simulink subsystem "sensorModel"  (R2021a)
settings: Solver=VariableStepAuto  StartTime=0.0  StopTime=10.0  RelTol=1e-3
settings Model: Creator=Laura  LastModifiedBy=Laura

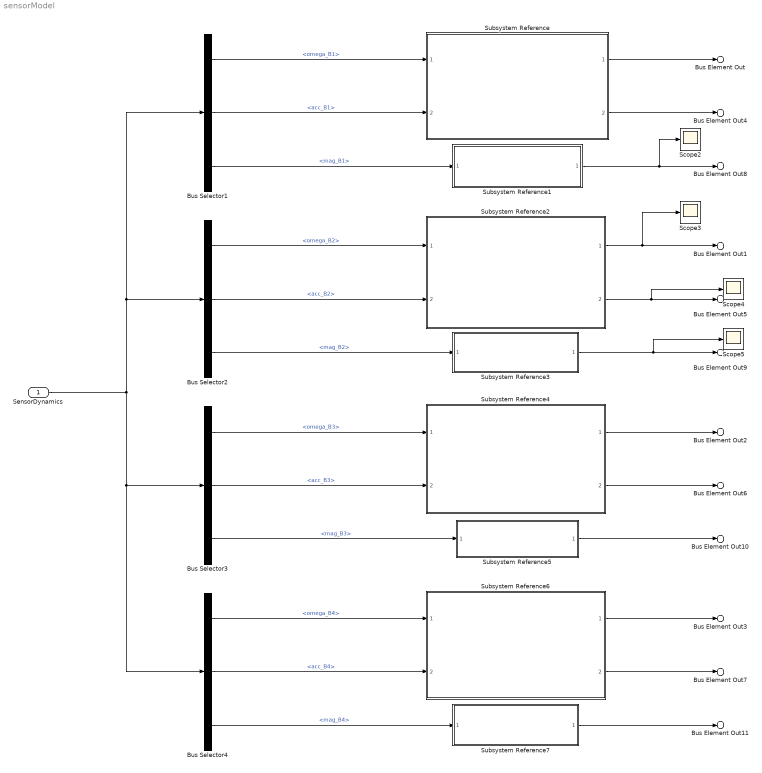
== system sensorModel ==
  SensorDynamics : Inport
  Bus Selector1 : BusSelector  OutputSignals=omega_B1,acc_B1,mag_B1
  Bus Selector2 : BusSelector  OutputSignals=omega_B2,acc_B2,mag_B2
  Bus Selector3 : BusSelector  OutputSignals=omega_B3,acc_B3,mag_B3
  Bus Selector4 : BusSelector  OutputSignals=omega_B4,acc_B4,mag_B4
  Scope{2..5} (4 alike) : Scope
  Subsystem Reference : Subsystem  ReferencedSubsystem=IMU1
  Subsystem Reference1 : Subsystem  ReferencedSubsystem=Magneto1
  Subsystem Reference2 : Subsystem  ReferencedSubsystem=IMU2
  Subsystem Reference3 : Subsystem  ReferencedSubsystem=Magneto2
  Subsystem Reference4 : Subsystem  ReferencedSubsystem=IMU3
  Subsystem Reference5 : Subsystem  ReferencedSubsystem=Magneto3
  Subsystem Reference6 : Subsystem  ReferencedSubsystem=IMU4
  Subsystem Reference7 : Subsystem  ReferencedSubsystem=Magneto4
  Bus Element Out : Outport  PortName=SensorData  Element=omega_B1_meas
  Bus Element Out1 : Outport  PortName=SensorData  Element=omega_B2_meas
  Bus Element Out2 : Outport  PortName=SensorData  Element=omega_B3_meas
  Bus Element Out3 : Outport  PortName=SensorData  Element=omega_B4_meas
  Bus Element Out4 : Outport  PortName=SensorData  Element=acc_B1_meas
  Bus Element Out5 : Outport  PortName=SensorData  Element=acc_B2_meas
  Bus Element Out6 : Outport  PortName=SensorData  Element=acc_B3_meas
  Bus Element Out7 : Outport  PortName=SensorData  Element=acc_B4_meas
  Bus Element Out8 : Outport  PortName=SensorData  Element=mag_B1_meas
  Bus Element Out9 : Outport  PortName=SensorData  Element=mag_B2_meas
  Bus Element Out10 : Outport  PortName=SensorData  Element=mag_B3_meas
  Bus Element Out11 : Outport  PortName=SensorData  Element=mag_B4_meas
  wires:
  SensorDynamics/1 -> Bus Selector3/1, Bus Selector4/1, Bus Selector1/1, Bus Selector2/1
  Bus Selector2/2 -> Subsystem Reference2/2  "<acc_B2>"
  Bus Selector2/1 -> Subsystem Reference2/1  "<omega_B2>"
  Subsystem Reference2/1 -> Bus Element Out1/1, Scope3/1
  Subsystem Reference2/2 -> Bus Element Out5/1, Scope4/1
  Bus Selector2/3 -> Subsystem Reference3/1  "<mag_B2>"
  Bus Selector4/3 -> Subsystem Reference7/1  "<mag_B4>"
  Bus Selector3/2 -> Subsystem Reference4/2  "<acc_B3>"
  Bus Selector3/1 -> Subsystem Reference4/1  "<omega_B3>"
  Bus Selector4/2 -> Subsystem Reference6/2  "<acc_B4>"
  Bus Selector4/1 -> Subsystem Reference6/1  "<omega_B4>"
  Bus Selector3/3 -> Subsystem Reference5/1  "<mag_B3>"
  Subsystem Reference4/1 -> Bus Element Out2/1
  Subsystem Reference6/1 -> Bus Element Out3/1
  Subsystem Reference4/2 -> Bus Element Out6/1
  Subsystem Reference5/1 -> Bus Element Out10/1
  Subsystem Reference6/2 -> Bus Element Out7/1
  Subsystem Reference7/1 -> Bus Element Out11/1
  Subsystem Reference3/1 -> Bus Element Out9/1, Scope5/1
  Subsystem Reference/2 -> Bus Element Out4/1
  Subsystem Reference/1 -> Bus Element Out/1
  Bus Selector1/1 -> Subsystem Reference/1  "<omega_B1>"
  Bus Selector1/2 -> Subsystem Reference/2  "<acc_B1>"
  Bus Selector1/3 -> Subsystem Reference1/1  "<mag_B1>"
  Subsystem Reference1/1 -> Bus Element Out8/1, Scope2/1
